simulink model "model"  (R2021a)
settings: Solver=ode4  StartTime=0.0  StopTime=sim_time  FixedStep=0.001  RelTol=1e-3
values from neighbouring files (symbols this model uses):
  ABS_ON = 0    [initialization.m]    (also in result_analysis.m = 1)
  Af = 2.36    [initialization.m]
  battery_capacity = 58*3.6*10^6    (= 208800000)    [initialization.m]
  battery_limit = 99    [initialization.m]
  brake_start = 10    [initialization.m]    (also in result_analysis.m)
  brakes = 1    [initialization.m]    (also in result_analysis.m)
  Cm = 310    [initialization.m]
  Cx = 0.27    [initialization.m]
  EBD_ON = 0    [initialization.m]    (also in result_analysis.m = 1)
  eta = 0.90    (= 0.9)    [initialization.m]
  Fx_lim = m*30    (= 54360)    [initialization.m]
  Fz = m*g/2    (= 8887.86)    [initialization.m]
  Gr = 10.5    [initialization.m]
  h = 0.55    [initialization.m]
  Ir = 1    [initialization.m]
  L = 2.77    [initialization.m]
  m = 1812    [initialization.m]
  mu = 0.5    [initialization.m]    (also in result_analysis.m)
  Pacn = Pace'    [initialization.m]
  pedal = 1    [initialization.m]    (also in result_analysis.m)
  phi = 0.95    [initialization.m]
  Pmax = 150000    [initialization.m]
  R = (D+2*H)/(2*1000)    (= 0.3488)    [initialization.m]
  regTorque = -0.1*g*R*m/(Gr)    (= -59.0492489143)    [initialization.m]
  rho = 1.225    [initialization.m]
  sim_time = 50    [initialization.m]    (also in result_analysis.m = 30)
  TCS_ON = 1    [initialization.m]    (also in result_analysis.m = 0)
  velstart = 0.5    [initialization.m]    (also in result_analysis.m = 30)
libraries: pid_lib x4
(part 2 of 2)

== matlab function model/Long Dynamics/MATLAB Function ==
  data: u input; y output
function y = fcn(u)
      if u <= 0
          y = 1;
      else
          y = 0;
      end
end

== matlab function model/Braking System/ABS controller/MATLAB Function ==
  data: v input; req_w output
function req_w= fcn(v)
R = 0.3488;
req_w = ( -0.1*v + v)/R; %

== matlab function model/Braking System/ABS controller/MATLAB Function2 ==
  data: brakes input; Fx input; ratio input; R input; u input size=[2,1]; Cf_f output; Cf_r output; s input size=[2,1]; v input; flag_f input; flag_front output size=1; flag_r input; flag_rear output size=1
function [Cf_f,Cf_r,flag_front,flag_rear] = fcn(brakes,Fx,ratio,R,u,s, v, flag_f,flag_r)
flag_front = flag_f;
flag_rear = flag_r;

%%signal that ABS is activated
if s(1) <= -0.2 
    flag_front = 1;
end
if s(2) <= -0.2 
    flag_rear = 1;
end

if s(1) >= -0.1
    flag_front = 0;
end
if s(2) >= -0.1
    flag_rear = 0;
end
%% apply brake torque
if flag_front == 1 && v>2.78
    Cf_f = u(1);
else 
    Cf_f = brakes*Fx*ratio(1)*R;
    %Cf_f = u(1);
end

if flag_rear == 1 && v>2.78
    Cf_r = u(2);
else 
    Cf_r = brakes*Fx*ratio(2)*R;
end

== matlab function model/Braking System/ABS controller/MATLAB Function1 ==
  data: Cf_r output; u input; Cm output; regTorque input
function [Cf_r,Cm] = fcn(u, regTorque)

if u >= abs(regTorque);
    %Cf_r = u;
    %Cm = -59.0492*0.5*0.95*10.5;
    Cf_r = (u - abs(regTorque))/2;
    Cm = 0;
else
    Cf_r = 0;
    Cm = u-abs(regTorque);
end

end

== matlab function model/Tracition Control System/TCS controller/MATLAB Function ==
  data: v input; req_w output
function req_w= fcn(v)
R = 0.3488;
req_w =(0.1*v + v)/R;

== matlab function model/torque generator/MATLAB Function ==
  data: reg input; battery_limit input; y output; SoC input
function y = fcn(reg,battery_limit, SoC)
if SoC < battery_limit
    y = reg;
else
    y = 0;
end

== matlab function model/Tracition Control System/TCS controller/MATLAB Function2 ==
  data: pedal input; R input; u input size=1; Cm_tcs output; s input size=1; flag_r input; flag_rear output size=1
function [Cm_tcs,flag_rear] = fcn(pedal,R,u,s,flag_r)



flag_rear = flag_r;

%%signal that TCS is activated
if abs(s) >= 0.2
    flag_rear = 1;
end


if abs(s) <= 0.1 
    flag_rear = 0;
end

%% apply brake torque
if flag_rear == 1 
    Cm_tcs = u;
else 
    Cm_tcs  = pedal*310;
end

== matlab function model/Braking System/MATLAB Function ==
  data: Cm_abs_in input; SoC input; Cm_abs_out output; battery_limit input
function Cm_abs_out = fcn(Cm_abs_in, SoC, battery_limit)

if SoC < battery_limit
    Cm_abs_out = Cm_abs_in;
else
    Cm_abs_out = 0;
end

== matlab function model/Braking System/ABS controller/EBD ==
  data: s_r input; y output; s_f input; v input
function y = fcn(s_r,s_f,v)
R = 0.3488;
if abs(s_r) > abs(s_f)
    y = (0.9*s_f*v + v)/R;
else
    y = 0;
end

== matlab function model/Tyre Rl/wheel dynamics FL3/MATLAB Function ==
  data: Fz input; v input; rr output
function rr = fcn(Fz,v)
    f0 = 0.009;
    f1 = 6.5e-6;
    rr = Fz*(f0 + f1*v^2);
end

== matlab function model/Tyre Rl/Pacejka 1 ==
  settings: fimath=|
      | fimath(...
      | 'RoundMode', 'floor',...
      | 'OverflowMode', 'wrap',...
      | 'ProductMode', 'KeepLSB', 'ProductWordLength', 32,...
      | 'SumMode', 'KeepLSB', 'SumWordLength', 32,...
      | 'CastBeforeSum', false)
  data: Pac input; gamma input; slip input; alfa input; Fz input; F_pac output; mu input; Vcx input; C_F output; R0 input
function [F_pac,C_F] = fcn(Pac,gamma,slip,alfa,Fz,mu,Vcx,R0)
% function for computing forces Fx, Fy and self-aligning torque Mz

% Pac   -> model structure with coeff. Pacejka 96
% slip  -> slip ratio [-] (-1:1)
% alfa  -> slip angle [rad]
% gamma -> camber [rad]
% Vcx,y velocity components of tire contact point C

% Structure building: Pacejka model coefficients
Pa_FZ0_ = Pac(1);
Pa_LFZ0 = Pac(2);
Pa_LmuV = Pac(3);
Pa_LKXK = Pac(4);
Pa_LKYA = Pac(5);
Pa_LCX_ = Pac(6);
Pa_LCY_ = Pac(7);
Pa_LEX_ = Pac(8);
Pa_LEY_ = Pac(9);
Pa_LHX_ = Pac(10);
Pa_LHY_ = Pac(11);
Pa_LVX_ = Pac(12);
Pa_LVY_ = Pac(13);
Pa_LKYG = Pac(14);
Pa_LKZG = Pac(15);
Pa_LT__ = Pac(16);
Pa_MR__ = Pac(17);
Pa_LXA_ = Pac(18);
Pa_LYK_ = Pac(19);
Pa_LVYK = Pac(20);
Pa_LS__ = Pac(21);
Pa_LCZ_ = Pac(22);
Pa_LMX_ = Pac(23);
Pa_LMY_ = Pac(24);
Pa_PCX1 = Pac(25);
Pa_PDX1 = Pac(26);
Pa_PDX2 = Pac(27);
Pa_PEX1 = Pac(28);
Pa_PEX2 = Pac(29);
Pa_PEX3 = Pac(30);
Pa_PEX4 = Pac(31);
Pa_PKX1 = Pac(32);
Pa_PKX2 = Pac(33);
Pa_PKX3 = Pac(34);
Pa_PHX1 = Pac(35);
Pa_PHX2 = Pac(36);
Pa_PVX1 = Pac(37);
Pa_PVX2 = Pac(38);
Pa_RBX1 = Pac(39);
Pa_RBX2 = Pac(40);
Pa_RCX1 = Pac(41);
Pa_RHX1 = Pac(42);
Pa_RTX1 = Pac(43);
Pa_RTX2 = Pac(44);
Pa_RTX3 = Pac(45);
Pa_QSX1 = Pac(46);
Pa_QSX2 = Pac(47);
Pa_QSX3 = Pac(48);
Pa_PCY1 = Pac(49);
Pa_PDY1 = Pac(50);
Pa_PDY2 = Pac(51);
Pa_PDY3 = Pac(52);
Pa_PEY1 = Pac(53);
Pa_PEY2 = Pac(54);
Pa_PEY3 = Pac(55);
Pa_PEY4 = Pac(56);
Pa_PKY1 = Pac(57);
Pa_PKY2 = Pac(58);
Pa_PKY3 = Pac(59);
Pa_PHY1 = Pac(60);
Pa_PHY2 = Pac(61);
Pa_PHY3 = Pac(62);
Pa_PVY1 = Pac(63);
Pa_PVY2 = Pac(64);
Pa_PVY3 = Pac(65);
Pa_PVY4 = Pac(66);
Pa_RBY1 = Pac(67);
Pa_RBY2 = Pac(68);
Pa_RBY3 = Pac(69);
Pa_RCY1 = Pac(70);
Pa_RHY1 = Pac(71);
Pa_RVY1 = Pac(72);
Pa_RVY2 = Pac(73);
Pa_RVY3 = Pac(74);
Pa_RVY4 = Pac(75);
Pa_RVY5 = Pac(76);
Pa_RVY6 = Pac(77);
Pa_PTY1 = Pac(78);
Pa_PTY2 = Pac(79);
Pa_QSY1 = Pac(80);
Pa_QSY2 = Pac(81);
Pa_QBZ1 = Pac(82);
Pa_QBZ2 = Pac(83);
Pa_QBZ3 = Pac(84);
Pa_QBZ4 = Pac(85);
Pa_QBZ5 = Pac(86);
Pa_QBZ6 = Pac(87);
Pa_QBZ9 = Pac(88);
Pa_QBZZ = Pac(89);
Pa_QCZ1 = Pac(90);
Pa_QDZ1 = Pac(91);
Pa_QDZ2 = Pac(92);
Pa_QDZ3 = Pac(93);
Pa_QDZ4 = Pac(94);
Pa_QDZ6 = Pac(95);
Pa_QDZ7 = Pac(96);
Pa_QDZ8 = Pac(97);
Pa_QDZ9 = Pac(98);
Pa_QEZ1 = Pac(99);
Pa_QEZ2 = Pac(100);
Pa_QEZ3 = Pac(101);
Pa_QEZ4 = Pac(102);
Pa_QEZ5 = Pac(103);
Pa_QHZ1 = Pac(104);
Pa_QHZ2 = Pac(105);
Pa_QHZ3 = Pac(106);
Pa_QHZ4 = Pac(107);
Pa_SSZ1 = Pac(108);
Pa_SSZ2 = Pac(109);
Pa_SSZ3 = Pac(110);
Pa_SSZ4 = Pac(111);
Pa_QTZ1 = Pac(112);

% Costants
epsi = 0.01;
eps_V = 0.1;
csi_0=1;
csi_4=1;
Amu = 10;
Pa_LmuX = mu;
Pa_LmuY = mu;

%-------------------------------- Fx pure slip ---------------------------
Cx = Pa_PCX1*Pa_LCX_;
dfz = (Fz-Pa_LFZ0*Pa_FZ0_)/(Pa_LFZ0*Pa_FZ0_);
mux = Pa_LmuX * (Pa_PDX1 + Pa_PDX2 * dfz);
Dx = mux*Fz; %*csi_1, con csi_1=1
%Shx = (Pa_PHX1+Pa_PHX2*dfz)*Pa_LHX_;
Shx = 0;
Kx = slip + Shx;
Ex = (Pa_PEX1+Pa_PEX2*dfz+Pa_PEX3*dfz^2)*(1-Pa_PEX4*sign(Kx))*Pa_LEX_;
if Ex>1 Et=1; end
Kxk = Fz*(Pa_PKX1+Pa_PKX2*dfz)*exp(Pa_PKX3*dfz)*Pa_LKXK;
Bx = Kxk/(Cx*Dx+epsi);
lam_mux  = Pa_LmuX*Amu/(1+(Amu-1)*Pa_LmuX);
SVx = Fz*(Pa_PVX1+Pa_PVX2*dfz)*(abs(Vcx)/(abs(Vcx)+eps_V))*Pa_LVX_*lam_mux; %*csi_1, con csi_1=1

% logitudinal slip stiffness (Fx slope in the origin)
C_Fk = Bx*Cx*Dx;

% longitudinal force
Fx0 = Dx*sin(Cx*atan(Bx*Kx-Ex*(Bx*Kx-atan(Bx*Kx)))) + SVx;

%---------------------------- Fy pure side slip --------------------------
seg=sign(Vcx);
if seg==0 seg=1; end
alfa_star = tan(alfa)*seg;
gam_star = sin(gamma);
Shy = (Pa_PHY1+Pa_PHY2*dfz)*Pa_LHY_+Pa_PHY3*gam_star*Pa_LKYG*csi_0+csi_4-1;
alfa_y = alfa_star + Shy;
Cy = Pa_PCY1*Pa_LCY_;
muy = Pa_LmuY*(Pa_PDY1+Pa_PDY2*dfz)*(1-Pa_PDY3*gam_star^2);
Dy = muy*Fz; %*csi_2, con csi_2=1
Ey = (Pa_PEY1+Pa_PEY2*dfz)*(1-(Pa_PEY3+Pa_PEY4*gam_star)*sign(alfa_y))*Pa_LEY_;
if Ey>1 Ey=1; end
Kya0 = Pa_PKY1*Pa_LFZ0*Pa_FZ0_*sin(2*atan(Fz/(Pa_PKY2*Pa_LFZ0*Pa_FZ0_)))*Pa_LKYA;
Kya = Kya0*(1-Pa_PKY3*gam_star^2); %*csi_3, con csi_3=1
By = Kya/(Cy*Dy+epsi);
lam_muy = Pa_LmuY*Amu/(1+(Amu-1)*Pa_LmuY);
SVy = Fz*((Pa_PVY1+Pa_PVY2*dfz)*Pa_LVY_+(Pa_PVY3+Pa_PVY4*dfz)*gam_star*Pa_LKYG )*lam_muy; %*csi_2, con csi_2=1
Kyg0 = (Pa_PHY3*Kya0+Fz*(Pa_PVY3+Pa_PVY4*dfz))*Pa_LKYG;

% cornering stiffness (Fy slope in the origin)
C_Fa = By*Cy*Dy;

% lateral force
Fy0 = Dy*sin(Cy*atan(By*alfa_y-Ey*(By*alfa_y-atan(By*alfa_y)))) + SVy;

% --------------------- Fx combined slip ------------------------------
Shxa = Pa_RHX1;
%Exa = Pa_REX1+Pa_REX2*dfz; NON esiste Pa.REX1 ne' Pa.REX2
Exa = 0;
Cxa = Pa_RCX1;
Bxa = Pa_RBX1*cos(atan(Pa_RBX2*slip))*Pa_LXA_;
alfaS = alfa_star+Shxa;
Gxa0 = cos(Cxa*atan(Bxa*Shxa-Exa*(Bxa*Shxa-atan(Bxa*Shxa))));
Gxa = cos(Cxa*atan(Bxa*alfaS-Exa*(Bxa*alfaS-atan(Bxa*alfaS))))/Gxa0;
Fx = Fx0*Gxa;

% ---------------------- Fy combined slip ------------------------------
Dvyk = muy*Fz*(Pa_RVY1+Pa_RVY2*dfz+Pa_RVY3*gam_star)*cos(atan(Pa_RVY4*alfa_star));%*csi_2, con csi_2=1
Svyk = Dvyk*sin(Pa_RVY5*atan(Pa_RVY6*slip));
Shyk = Pa_RHY1; %+Pa.RHY2*dfz; NON esiste Pa.RHY2
Cyk = Pa_RCY1;
Byk = Pa_RBY1*cos(atan(Pa_RBY2*(alfa_star-Pa_RBY3)))*Pa_LYK_;
%Eyk = Pa_REY1+Pa_REY2*dfz; NON esiste Pa.REY1 ne' Pa.REY2
Eyk = 0;
ks = slip+Shyk;
Gyk0 = cos(Cyk*atan(Byk*Shyk-Eyk*(Byk*Shyk-atan(Byk*Shyk))));
Gyk = cos(Cyk*atan(Byk*ks-Eyk*(Byk*ks-atan(Byk*ks))))/Gyk0;
Fy = Fy0*Gyk+Svyk;

% --------------------- Mz pure side slip  ---------------------------
Shf = Shy+SVy/Kya;
alfa_r = alfa_star+Shf;
Br = (Pa_QBZ9/Pa_LmuY+Pa_QBZZ*By*Cy); %*csi_6, con csi_6=1
%%% Pa_QBZZ e' in realta' QBZ10 scritto cosi' x ragioni di spazio
Cr = 1; %*csi_7, con csi_7=1
Dr = Fz*R0*((Pa_QDZ6+Pa_QDZ7*dfz)+(Pa_QDZ8+Pa_QDZ9*dfz)*gam_star)*cos(alfa)*Pa_LmuY*seg; %+csi_8-1, con csi_8=1
Mzr0 = Dr*cos(Cr*atan(Br*alfa_r));
Sht = Pa_QHZ1+Pa_QHZ2*dfz+(Pa_QHZ3+Pa_QHZ4*dfz)*gam_star;
alfa_t = alfa_star+Sht;
Bt = (Pa_QBZ1+Pa_QBZ2*dfz+Pa_QBZ3*dfz^2)*(1+Pa_QBZ5*abs(gam_star)+Pa_QBZ6*gam_star^2)*Pa_LKYA/Pa_LmuY;
if Bt<0 Bt=0; end
Ct = Pa_QCZ1;
Dt0 = Fz*R0/(Pa_LFZ0*Pa_FZ0_)*(Pa_QDZ1+Pa_QDZ2*dfz)*seg;
Dt = Dt0*(1+Pa_QDZ3*abs(gam_star)+Pa_QDZ4*gam_star^2); %*csi_5, con csi_5=1
Et = (Pa_QEZ1+Pa_QEZ2*dfz+Pa_QEZ3*dfz^2)*(1+(Pa_QEZ4+Pa_QEZ5*gam_star)*2/pi*atan(Bt*Ct*alfa_t));
if Et>1 Et=1; end
t0 = Dt*cos(Ct*atan(Bt*alfa_t - Et*(Bt*alfa_t-atan(Bt*alfa_t))))*cos(alfa);
Mz0 = -t0*Fy;
Kza0 = Dt0*Kya0;
%Kzg0 = Fz*R0*(Pa_QDZ8+Pa_QDZ9*dfz)-Dt0*Kyg0;

% aligning torque
Mz = Mz0 + Mzr0;

% ------------------------ Mz Combined -----------------------------
eps_k = 0; % 
lambda_s = Pa_LS__ ;
Fz0p = Pa_LFZ0*Pa_FZ0_;
K_yap = Kya + eps_k;
alfa_req = sqrt(alfa_r^2+(Kxk/K_yap)^2*slip^2)*sign(alfa_r);
alfa_teq = sqrt(alfa_t^2+(Kxk/K_yap)^2*slip^2)*sign(alfa_t);
s = R0*(Pa_SSZ1 + Pa_SSZ2*(Fy/Fz0p) + (Pa_SSZ3+Pa_SSZ4*dfz)*gam_star)*lambda_s;
Mzr = Dr*cos(Cr*atan(Br*alfa_req));
Fyp = Fy-Svyk; 
t = Dt*cos(Ct*atan(Bt*alfa_teq - Et*(Bt*alfa_teq-atan(Bt*alfa_teq))))*cos(alfa);
Mzp = -t*Fyp;
% aligning torque
Mz = Mzp + Mzr + s*Fx;
%%%%%%%%%%%%%%%%%%%%%%%

% Check that Fz is positive
if Fz <= 0
    Fx = 0;
    Fy = 0;
    Mz = 0;
end

% Output
F_pac = [Fx; Fy; Mz];
C_F = [C_Fk; C_Fa];

== matlab function model/Tyre Rr/SLIP RATIO ==
  data: v input; s output; vw input
function s = fcn(v,vw)
    
    s = (vw - v)/v;

== matlab function model/Tyre Rr/Pacejka 1 ==
  settings: fimath=|
      | fimath(...
      | 'RoundMode', 'floor',...
      | 'OverflowMode', 'wrap',...
      | 'ProductMode', 'KeepLSB', 'ProductWordLength', 32,...
      | 'SumMode', 'KeepLSB', 'SumWordLength', 32,...
      | 'CastBeforeSum', false)
  data: Pac input; gamma input; slip input; alfa input; Fz input; F_pac output; mu input; Vcx input; C_F output; R0 input
function [F_pac,C_F] = fcn(Pac,gamma,slip,alfa,Fz,mu,Vcx,R0)
% function for computing forces Fx, Fy and self-aligning torque Mz

% Pac   -> model structure with coeff. Pacejka 96
% slip  -> slip ratio [-] (-1:1)
% alfa  -> slip angle [rad]
% gamma -> camber [rad]
% Vcx,y velocity components of tire contact point C

% Structure building: Pacejka model coefficients
Pa_FZ0_ = Pac(1);
Pa_LFZ0 = Pac(2);
Pa_LmuV = Pac(3);
Pa_LKXK = Pac(4);
Pa_LKYA = Pac(5);
Pa_LCX_ = Pac(6);
Pa_LCY_ = Pac(7);
Pa_LEX_ = Pac(8);
Pa_LEY_ = Pac(9);
Pa_LHX_ = Pac(10);
Pa_LHY_ = Pac(11);
Pa_LVX_ = Pac(12);
Pa_LVY_ = Pac(13);
Pa_LKYG = Pac(14);
Pa_LKZG = Pac(15);
Pa_LT__ = Pac(16);
Pa_MR__ = Pac(17);
Pa_LXA_ = Pac(18);
Pa_LYK_ = Pac(19);
Pa_LVYK = Pac(20);
Pa_LS__ = Pac(21);
Pa_LCZ_ = Pac(22);
Pa_LMX_ = Pac(23);
Pa_LMY_ = Pac(24);
Pa_PCX1 = Pac(25);
Pa_PDX1 = Pac(26);
Pa_PDX2 = Pac(27);
Pa_PEX1 = Pac(28);
Pa_PEX2 = Pac(29);
Pa_PEX3 = Pac(30);
Pa_PEX4 = Pac(31);
Pa_PKX1 = Pac(32);
Pa_PKX2 = Pac(33);
Pa_PKX3 = Pac(34);
Pa_PHX1 = Pac(35);
Pa_PHX2 = Pac(36);
Pa_PVX1 = Pac(37);
Pa_PVX2 = Pac(38);
Pa_RBX1 = Pac(39);
Pa_RBX2 = Pac(40);
Pa_RCX1 = Pac(41);
Pa_RHX1 = Pac(42);
Pa_RTX1 = Pac(43);
Pa_RTX2 = Pac(44);
Pa_RTX3 = Pac(45);
Pa_QSX1 = Pac(46);
Pa_QSX2 = Pac(47);
Pa_QSX3 = Pac(48);
Pa_PCY1 = Pac(49);
Pa_PDY1 = Pac(50);
Pa_PDY2 = Pac(51);
Pa_PDY3 = Pac(52);
Pa_PEY1 = Pac(53);
Pa_PEY2 = Pac(54);
Pa_PEY3 = Pac(55);
Pa_PEY4 = Pac(56);
Pa_PKY1 = Pac(57);
Pa_PKY2 = Pac(58);
Pa_PKY3 = Pac(59);
Pa_PHY1 = Pac(60);
Pa_PHY2 = Pac(61);
Pa_PHY3 = Pac(62);
Pa_PVY1 = Pac(63);
Pa_PVY2 = Pac(64);
Pa_PVY3 = Pac(65);
Pa_PVY4 = Pac(66);
Pa_RBY1 = Pac(67);
Pa_RBY2 = Pac(68);
Pa_RBY3 = Pac(69);
Pa_RCY1 = Pac(70);
Pa_RHY1 = Pac(71);
Pa_RVY1 = Pac(72);
Pa_RVY2 = Pac(73);
Pa_RVY3 = Pac(74);
Pa_RVY4 = Pac(75);
Pa_RVY5 = Pac(76);
Pa_RVY6 = Pac(77);
Pa_PTY1 = Pac(78);
Pa_PTY2 = Pac(79);
Pa_QSY1 = Pac(80);
Pa_QSY2 = Pac(81);
Pa_QBZ1 = Pac(82);
Pa_QBZ2 = Pac(83);
Pa_QBZ3 = Pac(84);
Pa_QBZ4 = Pac(85);
Pa_QBZ5 = Pac(86);
Pa_QBZ6 = Pac(87);
Pa_QBZ9 = Pac(88);
Pa_QBZZ = Pac(89);
Pa_QCZ1 = Pac(90);
Pa_QDZ1 = Pac(91);
Pa_QDZ2 = Pac(92);
Pa_QDZ3 = Pac(93);
Pa_QDZ4 = Pac(94);
Pa_QDZ6 = Pac(95);
Pa_QDZ7 = Pac(96);
Pa_QDZ8 = Pac(97);
Pa_QDZ9 = Pac(98);
Pa_QEZ1 = Pac(99);
Pa_QEZ2 = Pac(100);
Pa_QEZ3 = Pac(101);
Pa_QEZ4 = Pac(102);
Pa_QEZ5 = Pac(103);
Pa_QHZ1 = Pac(104);
Pa_QHZ2 = Pac(105);
Pa_QHZ3 = Pac(106);
Pa_QHZ4 = Pac(107);
Pa_SSZ1 = Pac(108);
Pa_SSZ2 = Pac(109);
Pa_SSZ3 = Pac(110);
Pa_SSZ4 = Pac(111);
Pa_QTZ1 = Pac(112);

% Costants
epsi = 0.01;
eps_V = 0.1;
csi_0=1;
csi_4=1;
Amu = 10;
Pa_LmuX = mu;
Pa_LmuY = mu;

%-------------------------------- Fx pure slip ---------------------------
Cx = Pa_PCX1*Pa_LCX_;
dfz = (Fz-Pa_LFZ0*Pa_FZ0_)/(Pa_LFZ0*Pa_FZ0_);
mux = Pa_LmuX * (Pa_PDX1 + Pa_PDX2 * dfz);
Dx = mux*Fz; %*csi_1, con csi_1=1
%Shx = (Pa_PHX1+Pa_PHX2*dfz)*Pa_LHX_;
Shx = 0;
Kx = slip + Shx;
Ex = (Pa_PEX1+Pa_PEX2*dfz+Pa_PEX3*dfz^2)*(1-Pa_PEX4*sign(Kx))*Pa_LEX_;
if Ex>1 Et=1; end
Kxk = Fz*(Pa_PKX1+Pa_PKX2*dfz)*exp(Pa_PKX3*dfz)*Pa_LKXK;
Bx = Kxk/(Cx*Dx+epsi);
lam_mux  = Pa_LmuX*Amu/(1+(Amu-1)*Pa_LmuX);
SVx = Fz*(Pa_PVX1+Pa_PVX2*dfz)*(abs(Vcx)/(abs(Vcx)+eps_V))*Pa_LVX_*lam_mux; %*csi_1, con csi_1=1

% logitudinal slip stiffness (Fx slope in the origin)
C_Fk = Bx*Cx*Dx;

% longitudinal force
Fx0 = Dx*sin(Cx*atan(Bx*Kx-Ex*(Bx*Kx-atan(Bx*Kx)))) + SVx;

%---------------------------- Fy pure side slip --------------------------
seg=sign(Vcx);
if seg==0 seg=1; end
alfa_star = tan(alfa)*seg;
gam_star = sin(gamma);
Shy = (Pa_PHY1+Pa_PHY2*dfz)*Pa_LHY_+Pa_PHY3*gam_star*Pa_LKYG*csi_0+csi_4-1;
alfa_y = alfa_star + Shy;
Cy = Pa_PCY1*Pa_LCY_;
muy = Pa_LmuY*(Pa_PDY1+Pa_PDY2*dfz)*(1-Pa_PDY3*gam_star^2);
Dy = muy*Fz; %*csi_2, con csi_2=1
Ey = (Pa_PEY1+Pa_PEY2*dfz)*(1-(Pa_PEY3+Pa_PEY4*gam_star)*sign(alfa_y))*Pa_LEY_;
if Ey>1 Ey=1; end
Kya0 = Pa_PKY1*Pa_LFZ0*Pa_FZ0_*sin(2*atan(Fz/(Pa_PKY2*Pa_LFZ0*Pa_FZ0_)))*Pa_LKYA;
Kya = Kya0*(1-Pa_PKY3*gam_star^2); %*csi_3, con csi_3=1
By = Kya/(Cy*Dy+epsi);
lam_muy = Pa_LmuY*Amu/(1+(Amu-1)*Pa_LmuY);
SVy = Fz*((Pa_PVY1+Pa_PVY2*dfz)*Pa_LVY_+(Pa_PVY3+Pa_PVY4*dfz)*gam_star*Pa_LKYG )*lam_muy; %*csi_2, con csi_2=1
Kyg0 = (Pa_PHY3*Kya0+Fz*(Pa_PVY3+Pa_PVY4*dfz))*Pa_LKYG;

% cornering stiffness (Fy slope in the origin)
C_Fa = By*Cy*Dy;

% lateral force
Fy0 = Dy*sin(Cy*atan(By*alfa_y-Ey*(By*alfa_y-atan(By*alfa_y)))) + SVy;

% --------------------- Fx combined slip ------------------------------
Shxa = Pa_RHX1;
%Exa = Pa_REX1+Pa_REX2*dfz; NON esiste Pa.REX1 ne' Pa.REX2
Exa = 0;
Cxa = Pa_RCX1;
Bxa = Pa_RBX1*cos(atan(Pa_RBX2*slip))*Pa_LXA_;
alfaS = alfa_star+Shxa;
Gxa0 = cos(Cxa*atan(Bxa*Shxa-Exa*(Bxa*Shxa-atan(Bxa*Shxa))));
Gxa = cos(Cxa*atan(Bxa*alfaS-Exa*(Bxa*alfaS-atan(Bxa*alfaS))))/Gxa0;
Fx = Fx0*Gxa;

% ---------------------- Fy combined slip ------------------------------
Dvyk = muy*Fz*(Pa_RVY1+Pa_RVY2*dfz+Pa_RVY3*gam_star)*cos(atan(Pa_RVY4*alfa_star));%*csi_2, con csi_2=1
Svyk = Dvyk*sin(Pa_RVY5*atan(Pa_RVY6*slip));
Shyk = Pa_RHY1; %+Pa.RHY2*dfz; NON esiste Pa.RHY2
Cyk = Pa_RCY1;
Byk = Pa_RBY1*cos(atan(Pa_RBY2*(alfa_star-Pa_RBY3)))*Pa_LYK_;
%Eyk = Pa_REY1+Pa_REY2*dfz; NON esiste Pa.REY1 ne' Pa.REY2
Eyk = 0;
ks = slip+Shyk;
Gyk0 = cos(Cyk*atan(Byk*Shyk-Eyk*(Byk*Shyk-atan(Byk*Shyk))));
Gyk = cos(Cyk*atan(Byk*ks-Eyk*(Byk*ks-atan(Byk*ks))))/Gyk0;
Fy = Fy0*Gyk+Svyk;

% --------------------- Mz pure side slip  ---------------------------
Shf = Shy+SVy/Kya;
alfa_r = alfa_star+Shf;
Br = (Pa_QBZ9/Pa_LmuY+Pa_QBZZ*By*Cy); %*csi_6, con csi_6=1
%%% Pa_QBZZ e' in realta' QBZ10 scritto cosi' x ragioni di spazio
Cr = 1; %*csi_7, con csi_7=1
Dr = Fz*R0*((Pa_QDZ6+Pa_QDZ7*dfz)+(Pa_QDZ8+Pa_QDZ9*dfz)*gam_star)*cos(alfa)*Pa_LmuY*seg; %+csi_8-1, con csi_8=1
Mzr0 = Dr*cos(Cr*atan(Br*alfa_r));
Sht = Pa_QHZ1+Pa_QHZ2*dfz+(Pa_QHZ3+Pa_QHZ4*dfz)*gam_star;
alfa_t = alfa_star+Sht;
Bt = (Pa_QBZ1+Pa_QBZ2*dfz+Pa_QBZ3*dfz^2)*(1+Pa_QBZ5*abs(gam_star)+Pa_QBZ6*gam_star^2)*Pa_LKYA/Pa_LmuY;
if Bt<0 Bt=0; end
Ct = Pa_QCZ1;
Dt0 = Fz*R0/(Pa_LFZ0*Pa_FZ0_)*(Pa_QDZ1+Pa_QDZ2*dfz)*seg;
Dt = Dt0*(1+Pa_QDZ3*abs(gam_star)+Pa_QDZ4*gam_star^2); %*csi_5, con csi_5=1
Et = (Pa_QEZ1+Pa_QEZ2*dfz+Pa_QEZ3*dfz^2)*(1+(Pa_QEZ4+Pa_QEZ5*gam_star)*2/pi*atan(Bt*Ct*alfa_t));
if Et>1 Et=1; end
t0 = Dt*cos(Ct*atan(Bt*alfa_t - Et*(Bt*alfa_t-atan(Bt*alfa_t))))*cos(alfa);
Mz0 = -t0*Fy;
Kza0 = Dt0*Kya0;
%Kzg0 = Fz*R0*(Pa_QDZ8+Pa_QDZ9*dfz)-Dt0*Kyg0;

% aligning torque
Mz = Mz0 + Mzr0;

% ------------------------ Mz Combined -----------------------------
eps_k = 0; % 
lambda_s = Pa_LS__ ;
Fz0p = Pa_LFZ0*Pa_FZ0_;
K_yap = Kya + eps_k;
alfa_req = sqrt(alfa_r^2+(Kxk/K_yap)^2*slip^2)*sign(alfa_r);
alfa_teq = sqrt(alfa_t^2+(Kxk/K_yap)^2*slip^2)*sign(alfa_t);
s = R0*(Pa_SSZ1 + Pa_SSZ2*(Fy/Fz0p) + (Pa_SSZ3+Pa_SSZ4*dfz)*gam_star)*lambda_s;
Mzr = Dr*cos(Cr*atan(Br*alfa_req));
Fyp = Fy-Svyk; 
t = Dt*cos(Ct*atan(Bt*alfa_teq - Et*(Bt*alfa_teq-atan(Bt*alfa_teq))))*cos(alfa);
Mzp = -t*Fyp;
% aligning torque
Mz = Mzp + Mzr + s*Fx;
%%%%%%%%%%%%%%%%%%%%%%%

% Check that Fz is positive
if Fz <= 0
    Fx = 0;
    Fy = 0;
    Mz = 0;
end

% Output
F_pac = [Fx; Fy; Mz];
C_F = [C_Fk; C_Fa];

== matlab function model/Tyre Rl/SLIP RATIO ==
  data: v input; s output; vw input
function s = fcn(v,vw)
    
    s = (vw - v)/v;

== matlab function model/Tyre Rr/wheel dynamics FL3/MATLAB Function ==
  data: Fz input; v input; rr output
function rr = fcn(Fz,v)
    f0 = 0.009;
    f1 = 6.5e-6;
    rr = Fz*(f0 + f1*v^2);
end

== matlab function model/Tyre Fl/Pacejka 1 ==
  settings: fimath=|
      | fimath(...
      | 'RoundMode', 'floor',...
      | 'OverflowMode', 'wrap',...
      | 'ProductMode', 'KeepLSB', 'ProductWordLength', 32,...
      | 'SumMode', 'KeepLSB', 'SumWordLength', 32,...
      | 'CastBeforeSum', false)
  data: Pac input; gamma input; slip input; alfa input; Fz input; F_pac output; mu input; Vcx input; C_F output; R0 input
function [F_pac,C_F] = fcn(Pac,gamma,slip,alfa,Fz,mu,Vcx,R0)
% function for computing forces Fx, Fy and self-aligning torque Mz

% Pac   -> model structure with coeff. Pacejka 96
% slip  -> slip ratio [-] (-1:1)
% alfa  -> slip angle [rad]
% gamma -> camber [rad]
% Vcx,y velocity components of tire contact point C

% Structure building: Pacejka model coefficients
Pa_FZ0_ = Pac(1);
Pa_LFZ0 = Pac(2);
Pa_LmuV = Pac(3);
Pa_LKXK = Pac(4);
Pa_LKYA = Pac(5);
Pa_LCX_ = Pac(6);
Pa_LCY_ = Pac(7);
Pa_LEX_ = Pac(8);
Pa_LEY_ = Pac(9);
Pa_LHX_ = Pac(10);
Pa_LHY_ = Pac(11);
Pa_LVX_ = Pac(12);
Pa_LVY_ = Pac(13);
Pa_LKYG = Pac(14);
Pa_LKZG = Pac(15);
Pa_LT__ = Pac(16);
Pa_MR__ = Pac(17);
Pa_LXA_ = Pac(18);
Pa_LYK_ = Pac(19);
Pa_LVYK = Pac(20);
Pa_LS__ = Pac(21);
Pa_LCZ_ = Pac(22);
Pa_LMX_ = Pac(23);
Pa_LMY_ = Pac(24);
Pa_PCX1 = Pac(25);
Pa_PDX1 = Pac(26);
Pa_PDX2 = Pac(27);
Pa_PEX1 = Pac(28);
Pa_PEX2 = Pac(29);
Pa_PEX3 = Pac(30);
Pa_PEX4 = Pac(31);
Pa_PKX1 = Pac(32);
Pa_PKX2 = Pac(33);
Pa_PKX3 = Pac(34);
Pa_PHX1 = Pac(35);
Pa_PHX2 = Pac(36);
Pa_PVX1 = Pac(37);
Pa_PVX2 = Pac(38);
Pa_RBX1 = Pac(39);
Pa_RBX2 = Pac(40);
Pa_RCX1 = Pac(41);
Pa_RHX1 = Pac(42);
Pa_RTX1 = Pac(43);
Pa_RTX2 = Pac(44);
Pa_RTX3 = Pac(45);
Pa_QSX1 = Pac(46);
Pa_QSX2 = Pac(47);
Pa_QSX3 = Pac(48);
Pa_PCY1 = Pac(49);
Pa_PDY1 = Pac(50);
Pa_PDY2 = Pac(51);
Pa_PDY3 = Pac(52);
Pa_PEY1 = Pac(53);
Pa_PEY2 = Pac(54);
Pa_PEY3 = Pac(55);
Pa_PEY4 = Pac(56);
Pa_PKY1 = Pac(57);
Pa_PKY2 = Pac(58);
Pa_PKY3 = Pac(59);
Pa_PHY1 = Pac(60);
Pa_PHY2 = Pac(61);
Pa_PHY3 = Pac(62);
Pa_PVY1 = Pac(63);
Pa_PVY2 = Pac(64);
Pa_PVY3 = Pac(65);
Pa_PVY4 = Pac(66);
Pa_RBY1 = Pac(67);
Pa_RBY2 = Pac(68);
Pa_RBY3 = Pac(69);
Pa_RCY1 = Pac(70);
Pa_RHY1 = Pac(71);
Pa_RVY1 = Pac(72);
Pa_RVY2 = Pac(73);
Pa_RVY3 = Pac(74);
Pa_RVY4 = Pac(75);
Pa_RVY5 = Pac(76);
Pa_RVY6 = Pac(77);
Pa_PTY1 = Pac(78);
Pa_PTY2 = Pac(79);
Pa_QSY1 = Pac(80);
Pa_QSY2 = Pac(81);
Pa_QBZ1 = Pac(82);
Pa_QBZ2 = Pac(83);
Pa_QBZ3 = Pac(84);
Pa_QBZ4 = Pac(85);
Pa_QBZ5 = Pac(86);
Pa_QBZ6 = Pac(87);
Pa_QBZ9 = Pac(88);
Pa_QBZZ = Pac(89);
Pa_QCZ1 = Pac(90);
Pa_QDZ1 = Pac(91);
Pa_QDZ2 = Pac(92);
Pa_QDZ3 = Pac(93);
Pa_QDZ4 = Pac(94);
Pa_QDZ6 = Pac(95);
Pa_QDZ7 = Pac(96);
Pa_QDZ8 = Pac(97);
Pa_QDZ9 = Pac(98);
Pa_QEZ1 = Pac(99);
Pa_QEZ2 = Pac(100);
Pa_QEZ3 = Pac(101);
Pa_QEZ4 = Pac(102);
Pa_QEZ5 = Pac(103);
Pa_QHZ1 = Pac(104);
Pa_QHZ2 = Pac(105);
Pa_QHZ3 = Pac(106);
Pa_QHZ4 = Pac(107);
Pa_SSZ1 = Pac(108);
Pa_SSZ2 = Pac(109);
Pa_SSZ3 = Pac(110);
Pa_SSZ4 = Pac(111);
Pa_QTZ1 = Pac(112);

% Costants
epsi = 0.01;
eps_V = 0.1;
csi_0=1;
csi_4=1;
Amu = 10;
Pa_LmuX = mu;
Pa_LmuY = mu;

%-------------------------------- Fx pure slip ---------------------------
Cx = Pa_PCX1*Pa_LCX_;
dfz = (Fz-Pa_LFZ0*Pa_FZ0_)/(Pa_LFZ0*Pa_FZ0_);
mux = Pa_LmuX * (Pa_PDX1 + Pa_PDX2 * dfz);
Dx = mux*Fz; %*csi_1, con csi_1=1
%Shx = (Pa_PHX1+Pa_PHX2*dfz)*Pa_LHX_;
Shx = 0;
Kx = slip + Shx;
Ex = (Pa_PEX1+Pa_PEX2*dfz+Pa_PEX3*dfz^2)*(1-Pa_PEX4*sign(Kx))*Pa_LEX_;
if Ex>1 Et=1; end
Kxk = Fz*(Pa_PKX1+Pa_PKX2*dfz)*exp(Pa_PKX3*dfz)*Pa_LKXK;
Bx = Kxk/(Cx*Dx+epsi);
lam_mux  = Pa_LmuX*Amu/(1+(Amu-1)*Pa_LmuX);
SVx = Fz*(Pa_PVX1+Pa_PVX2*dfz)*(abs(Vcx)/(abs(Vcx)+eps_V))*Pa_LVX_*lam_mux; %*csi_1, con csi_1=1

% logitudinal slip stiffness (Fx slope in the origin)
C_Fk = Bx*Cx*Dx;

% longitudinal force
Fx0 = Dx*sin(Cx*atan(Bx*Kx-Ex*(Bx*Kx-atan(Bx*Kx)))) + SVx;

%---------------------------- Fy pure side slip --------------------------
seg=sign(Vcx);
if seg==0 seg=1; end
alfa_star = tan(alfa)*seg;
gam_star = sin(gamma);
Shy = (Pa_PHY1+Pa_PHY2*dfz)*Pa_LHY_+Pa_PHY3*gam_star*Pa_LKYG*csi_0+csi_4-1;
alfa_y = alfa_star + Shy;
Cy = Pa_PCY1*Pa_LCY_;
muy = Pa_LmuY*(Pa_PDY1+Pa_PDY2*dfz)*(1-Pa_PDY3*gam_star^2);
Dy = muy*Fz; %*csi_2, con csi_2=1
Ey = (Pa_PEY1+Pa_PEY2*dfz)*(1-(Pa_PEY3+Pa_PEY4*gam_star)*sign(alfa_y))*Pa_LEY_;
if Ey>1 Ey=1; end
Kya0 = Pa_PKY1*Pa_LFZ0*Pa_FZ0_*sin(2*atan(Fz/(Pa_PKY2*Pa_LFZ0*Pa_FZ0_)))*Pa_LKYA;
Kya = Kya0*(1-Pa_PKY3*gam_star^2); %*csi_3, con csi_3=1
By = Kya/(Cy*Dy+epsi);
lam_muy = Pa_LmuY*Amu/(1+(Amu-1)*Pa_LmuY);
SVy = Fz*((Pa_PVY1+Pa_PVY2*dfz)*Pa_LVY_+(Pa_PVY3+Pa_PVY4*dfz)*gam_star*Pa_LKYG )*lam_muy; %*csi_2, con csi_2=1
Kyg0 = (Pa_PHY3*Kya0+Fz*(Pa_PVY3+Pa_PVY4*dfz))*Pa_LKYG;

% cornering stiffness (Fy slope in the origin)
C_Fa = By*Cy*Dy;

% lateral force
Fy0 = Dy*sin(Cy*atan(By*alfa_y-Ey*(By*alfa_y-atan(By*alfa_y)))) + SVy;

% --------------------- Fx combined slip ------------------------------
Shxa = Pa_RHX1;
%Exa = Pa_REX1+Pa_REX2*dfz; NON esiste Pa.REX1 ne' Pa.REX2
Exa = 0;
Cxa = Pa_RCX1;
Bxa = Pa_RBX1*cos(atan(Pa_RBX2*slip))*Pa_LXA_;
alfaS = alfa_star+Shxa;
Gxa0 = cos(Cxa*atan(Bxa*Shxa-Exa*(Bxa*Shxa-atan(Bxa*Shxa))));
Gxa = cos(Cxa*atan(Bxa*alfaS-Exa*(Bxa*alfaS-atan(Bxa*alfaS))))/Gxa0;
Fx = Fx0*Gxa;

% ---------------------- Fy combined slip ------------------------------
Dvyk = muy*Fz*(Pa_RVY1+Pa_RVY2*dfz+Pa_RVY3*gam_star)*cos(atan(Pa_RVY4*alfa_star));%*csi_2, con csi_2=1
Svyk = Dvyk*sin(Pa_RVY5*atan(Pa_RVY6*slip));
Shyk = Pa_RHY1; %+Pa.RHY2*dfz; NON esiste Pa.RHY2
Cyk = Pa_RCY1;
Byk = Pa_RBY1*cos(atan(Pa_RBY2*(alfa_star-Pa_RBY3)))*Pa_LYK_;
%Eyk = Pa_REY1+Pa_REY2*dfz; NON esiste Pa.REY1 ne' Pa.REY2
Eyk = 0;
ks = slip+Shyk;
Gyk0 = cos(Cyk*atan(Byk*Shyk-Eyk*(Byk*Shyk-atan(Byk*Shyk))));
Gyk = cos(Cyk*atan(Byk*ks-Eyk*(Byk*ks-atan(Byk*ks))))/Gyk0;
Fy = Fy0*Gyk+Svyk;

% --------------------- Mz pure side slip  ---------------------------
Shf = Shy+SVy/Kya;
alfa_r = alfa_star+Shf;
Br = (Pa_QBZ9/Pa_LmuY+Pa_QBZZ*By*Cy); %*csi_6, con csi_6=1
%%% Pa_QBZZ e' in realta' QBZ10 scritto cosi' x ragioni di spazio
Cr = 1; %*csi_7, con csi_7=1
Dr = Fz*R0*((Pa_QDZ6+Pa_QDZ7*dfz)+(Pa_QDZ8+Pa_QDZ9*dfz)*gam_star)*cos(alfa)*Pa_LmuY*seg; %+csi_8-1, con csi_8=1
Mzr0 = Dr*cos(Cr*atan(Br*alfa_r));
Sht = Pa_QHZ1+Pa_QHZ2*dfz+(Pa_QHZ3+Pa_QHZ4*dfz)*gam_star;
alfa_t = alfa_star+Sht;
Bt = (Pa_QBZ1+Pa_QBZ2*dfz+Pa_QBZ3*dfz^2)*(1+Pa_QBZ5*abs(gam_star)+Pa_QBZ6*gam_star^2)*Pa_LKYA/Pa_LmuY;
if Bt<0 Bt=0; end
Ct = Pa_QCZ1;
Dt0 = Fz*R0/(Pa_LFZ0*Pa_FZ0_)*(Pa_QDZ1+Pa_QDZ2*dfz)*seg;
Dt = Dt0*(1+Pa_QDZ3*abs(gam_star)+Pa_QDZ4*gam_star^2); %*csi_5, con csi_5=1
Et = (Pa_QEZ1+Pa_QEZ2*dfz+Pa_QEZ3*dfz^2)*(1+(Pa_QEZ4+Pa_QEZ5*gam_star)*2/pi*atan(Bt*Ct*alfa_t));
if Et>1 Et=1; end
t0 = Dt*cos(Ct*atan(Bt*alfa_t - Et*(Bt*alfa_t-atan(Bt*alfa_t))))*cos(alfa);
Mz0 = -t0*Fy;
Kza0 = Dt0*Kya0;
%Kzg0 = Fz*R0*(Pa_QDZ8+Pa_QDZ9*dfz)-Dt0*Kyg0;

% aligning torque
Mz = Mz0 + Mzr0;

% ------------------------ Mz Combined -----------------------------
eps_k = 0; % 
lambda_s = Pa_LS__ ;
Fz0p = Pa_LFZ0*Pa_FZ0_;
K_yap = Kya + eps_k;
alfa_req = sqrt(alfa_r^2+(Kxk/K_yap)^2*slip^2)*sign(alfa_r);
alfa_teq = sqrt(alfa_t^2+(Kxk/K_yap)^2*slip^2)*sign(alfa_t);
s = R0*(Pa_SSZ1 + Pa_SSZ2*(Fy/Fz0p) + (Pa_SSZ3+Pa_SSZ4*dfz)*gam_star)*lambda_s;
Mzr = Dr*cos(Cr*atan(Br*alfa_req));
Fyp = Fy-Svyk; 
t = Dt*cos(Ct*atan(Bt*alfa_teq - Et*(Bt*alfa_teq-atan(Bt*alfa_teq))))*cos(alfa);
Mzp = -t*Fyp;
% aligning torque
Mz = Mzp + Mzr + s*Fx;
%%%%%%%%%%%%%%%%%%%%%%%

% Check that Fz is positive
if Fz <= 0
    Fx = 0;
    Fy = 0;
    Mz = 0;
end

% Output
F_pac = [Fx; Fy; Mz];
C_F = [C_Fk; C_Fa];
